simulink model "Simulation_DOA_rearanged_2020a"  (R2020a)
settings: Solver=ode4  StartTime=0.0  StopTime=0.03  RelTol=1e-3
values from neighbouring files (symbols this model uses):
  f_range = [20e3 45e3]    [Init.m]
  FFT_LENGTH = 256    [Init.m]
  noise_on_off = false    [Init.m]
  noise_type = 1    [Init.m]
  Sampling_rate = 256e3    (= 256000)    [Init.m]
undefined symbols (not defined in the file or in its folder): Coeff_han, runSim
libraries: dspsigops x29, dspsrcs4 x16, dsphdlmathfun x4, dsphdlxfrm x4, simulink x2, hdlsllib x1
(part 1 of 2)
settings Model: Creator=tigro  LastModifiedBy=franc
settings OptimizationCC: BlockReduction=off  ConditionallyExecuteInputs=off  DefaultParameterBehavior=Inlined
settings DebuggingCC: AlgebraicLoopMsg=error  ParameterOverflowMsg=none
settings HardwareCC: ProdBitPerPointer=32  ProdBitPerSizeT=32  ProdBitPerPtrDiffT=32  ProdLargestAtomicFloat=None  ProdIntDivRoundTo=Undefined  ProdEndianess=Unspecified  ProdWordSize=32  ProdHWDeviceType=ASIC/FPGA->ASIC/FPGA  TargetBitPerPointer=64  TargetBitPerSizeT=64  TargetBitPerPtrDiffT=64  TargetLongLongMode=on  TargetIntDivRoundTo=Zero  TargetEndianess=LittleEndian  TargetWordSize=64  TargetHWDeviceType=Custom Processor->MATLAB Host Computer  ProdEqTarget=off

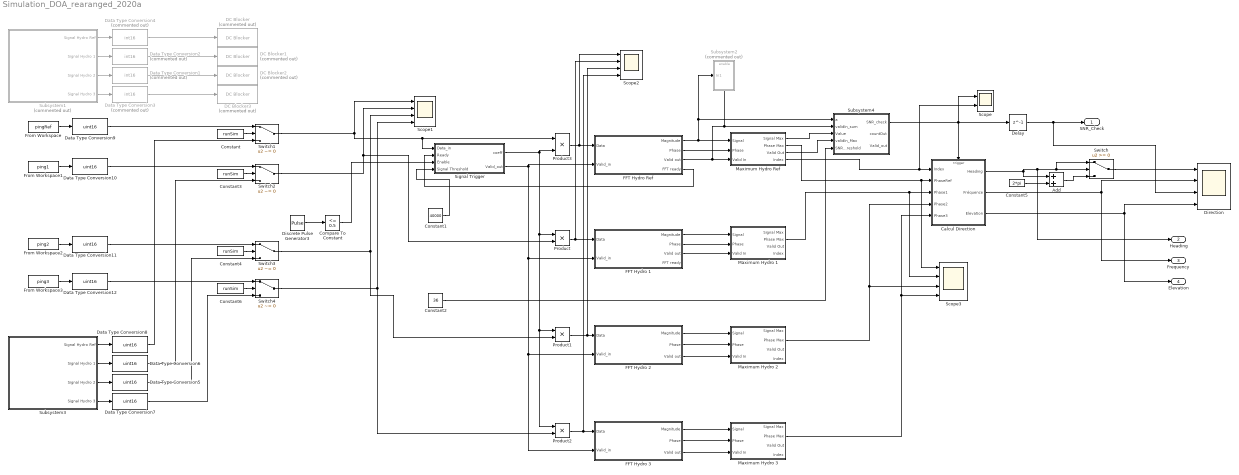
== system Simulation_DOA_rearanged_2020a ==
  Add : Sum
  Calcul Direction : Subsystem
  Compare To Constant : simulink/Logic and Bit Operations/Compare To Constant  relop=<=  const=0.5  OutDataTypeStr=boolean
  Constant{,3..4,6} (4 alike) : Constant  Value=runSim  SampleTime=-1
  Constant1 : Constant  Value=40000  OutDataTypeStr=uint16  SampleTime=-1
  Constant2 : Constant  Value=36  OutDataTypeStr=uint16  SampleTime=-1
  Constant5 : Constant  Value=2*pi
  DC Blocker{,1..3} (4 alike) : dspsigops/DC Blocker  Commented=on  Algorithm=FIR  NormalizedBandwidth=0.001  Length=50  Order=6  SimulateUsing=Code generation
      settings: SourceProductBaseCode=DS
  Data Type Conversion{1..4} (4 alike) : DataTypeConversion  Commented=on  OutMax=[4096]  OutDataTypeStr=int16
  Data Type Conversion{5..12} (8 alike) : DataTypeConversion  OutMax=[65535]  OutDataTypeStr=uint16
  Delay : Delay  DelayLength=1  InitialCondition=0
  Direction : Scope  NumInputPorts=4
  Discrete Pulse Generator3 : DiscretePulseGenerator  Period=512  PulseWidth=256  PhaseDelay=250  SampleTime=1/Sampling_rate
  FFT Hydro 1 : Subsystem
  FFT Hydro 2 : Subsystem
  FFT Hydro 3 : Subsystem
  FFT Hydro Ref : Subsystem
  From Workspace : FromWorkspace  VariableName=pingRef  SampleTime=1/Sampling_rate
  From Workspace1 : FromWorkspace  VariableName=ping1  SampleTime=1/Sampling_rate
  From Workspace2 : FromWorkspace  VariableName=ping2  SampleTime=1/Sampling_rate
  From Workspace3 : FromWorkspace  VariableName=ping3  SampleTime=1/Sampling_rate
  Maximum Hydro 1 : Subsystem
  Maximum Hydro 2 : Subsystem
  Maximum Hydro 3 : Subsystem
  Maximum Hydro Ref : Subsystem
  Product{,1..3} (4 alike) : Product
  Scope : Scope  NumInputPorts=2
  Scope1 : Scope  NumInputPorts=4
  Scope2 : Scope  NumInputPorts=4
  Scope3 : Scope  NumInputPorts=4
  Signal Trigger : Subsystem
  Subsystem1 : Subsystem  Commented=on
  Subsystem2 : Subsystem  Commented=on
  Subsystem3 : Subsystem
  Subsystem4 : Subsystem
  Switch : Switch
  Switch{1..4} (4 alike) : Switch  Criteria=u2 ~= 0
  SNR_Check : Outport
  Heading : Outport  Port=2
  Frequency : Outport  Port=3
  Elevation : Outport  Port=4
  wires:
  Maximum Hydro Ref/1(Signal Max) -> Subsystem4/3(" Value")
  Subsystem4/1(SNR_check) -> Delay/1, Scope/1, Calcul Direction/Trigger
  Maximum Hydro Ref/4(Index) -> Scope/2, Calcul Direction/1(Index)
  Calcul Direction/1(Heading) -> Heading/1, Switch/2, Switch/1, Add/1
  Add/1 -> Switch/3
  Constant5/1 -> Add/2
  Product3/1 -> Scope2/1, FFT Hydro Ref/1(Data)
  Product/1 -> Scope2/2, FFT Hydro 1/1(Data)
  Product1/1 -> Scope2/3, FFT Hydro 2/1(Data)
  Product2/1 -> Scope2/4, FFT Hydro 3/1(Data)
  FFT Hydro Ref/2(Phase) -> Maximum Hydro Ref/2(Phase)
  Maximum Hydro Ref/2(Phase Max) -> Scope3/1, Calcul Direction/2(PhaseRef)
  Maximum Hydro 1/2(Phase Max) -> Scope3/2, Calcul Direction/3(Phase1)
  Maximum Hydro 2/2(Phase Max) -> Calcul Direction/4(Phase2), Scope3/3
  Maximum Hydro 3/2(Phase Max) -> Calcul Direction/5(Phase3), Scope3/4
  Signal Trigger/2(Valid_out) -> FFT Hydro Ref/2(Valid_in), FFT Hydro 1/2(Valid_in), FFT Hydro 3/2(Valid_in), FFT Hydro 2/2(Valid_in)
  Signal Trigger/1(coeff) -> Product3/2, Product/1, Product1/1, Product2/1
  FFT Hydro 1/1(Magnitude) -> Maximum Hydro 1/1(Signal)
  FFT Hydro 1/2(Phase) -> Maximum Hydro 1/2(Phase)
  FFT Hydro 1/3(Valid out) -> Maximum Hydro 1/3(Valid In)
  FFT Hydro 2/1(Magnitude) -> Maximum Hydro 2/1(Signal)
  FFT Hydro 2/2(Phase) -> Maximum Hydro 2/2(Phase)
  FFT Hydro 2/3(Valid out) -> Maximum Hydro 2/3(Valid In)
  FFT Hydro 3/1(Magnitude) -> Maximum Hydro 3/1(Signal)
  FFT Hydro 3/2(Phase) -> Maximum Hydro 3/2(Phase)
  FFT Hydro 3/3(Valid out) -> Maximum Hydro 3/3(Valid In)
  Maximum Hydro Ref/3(Valid Out) -> Subsystem4/4(validIn_Max)
  FFT Hydro Ref/4(FFT ready) -> Signal Trigger/2(Ready)
  FFT Hydro Ref/3(Valid out) -> Maximum Hydro Ref/3(Valid In), Subsystem2/Enable, Subsystem4/2(validIn_sum)
  Calcul Direction/2(Fréquence) -> Frequency/1, Direction/2
  Switch/1 -> Direction/1
  FFT Hydro Ref/1(Magnitude) -> Maximum Hydro Ref/1(Signal), Subsystem2/1(In1), Subsystem4/1(a)
  Subsystem1/4(Signal Hydro 3) -> Data Type Conversion3/1
  Data Type Conversion3/1 -> DC Blocker3/1
  Data Type Conversion2/1 -> DC Blocker1/1
  Data Type Conversion4/1 -> DC Blocker/1
  Data Type Conversion1/1 -> DC Blocker2/1
  Subsystem1/2(Signal Hydro 1) -> Data Type Conversion2/1
  Subsystem1/3(Signal Hydro 2) -> Data Type Conversion1/1
  Subsystem1/1(Signal Hydro Ref) -> Data Type Conversion4/1
  Subsystem3/4(Signal Hydro 3) -> Data Type Conversion7/1
  Subsystem3/2(Signal Hydro 1) -> Data Type Conversion6/1
  Subsystem3/3(Signal Hydro 2) -> Data Type Conversion5/1
  Subsystem3/1(Signal Hydro Ref) -> Data Type Conversion8/1
  Switch2/1 -> Scope1/2, Product/2
  Switch3/1 -> Product1/2, Scope1/3
  Switch4/1 -> Product2/2, Scope1/4
  Discrete Pulse Generator3/1 -> Compare To Constant/1
  Switch1/1 -> Signal Trigger/1(Data_in), Product3/1, Scope1/1
  Delay/1 -> SNR_Check/1, Direction/3
  Compare To Constant/1 -> Signal Trigger/3(Enable)
  Constant1/1 -> Signal Trigger/4(Signal Threshold)
  Constant2/1 -> Subsystem4/5(SNR_Threshold)
  From Workspace/1 -> Data Type Conversion9/1
  From Workspace1/1 -> Data Type Conversion10/1
  From Workspace2/1 -> Data Type Conversion11/1
  From Workspace3/1 -> Data Type Conversion12/1
  Calcul Direction/3(Elevation) -> Elevation/1, Direction/4
  Data Type Conversion9/1 -> Switch1/1
  Data Type Conversion8/1 -> Switch1/3
  Data Type Conversion10/1 -> Switch2/1
  Data Type Conversion11/1 -> Switch3/1
  Data Type Conversion5/1 -> Switch3/3
  Data Type Conversion7/1 -> Switch4/3
  Data Type Conversion6/1 -> Switch2/3
  Data Type Conversion12/1 -> Switch4/1
  Constant/1 -> Switch1/2
  Constant3/1 -> Switch2/2
  Constant4/1 -> Switch3/2
  Constant6/1 -> Switch4/2

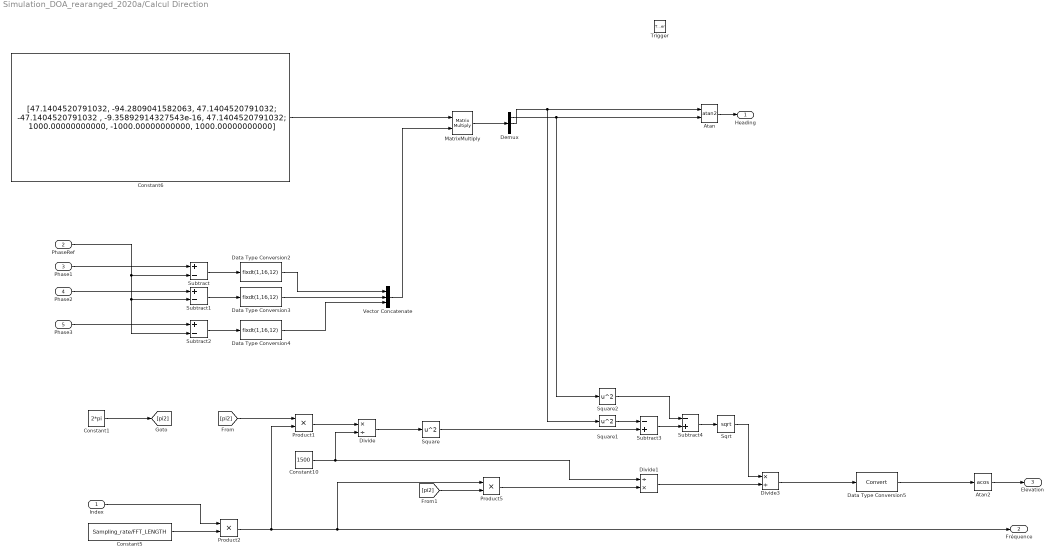
== system Simulation_DOA_rearanged_2020a/Calcul Direction ==
  Index : Inport
  PhaseRef : Inport  Port=2
  Phase1 : Inport  Port=3
  Phase2 : Inport  Port=4
  Phase3 : Inport  Port=5
  Trigger : TriggerPort  VariantControl=Variant  PortDimensions=1
  Atan : Trigonometry  Operator=atan2  ApproximationMethod=CORDIC  OutputSignalType=real
  Atan2 : Trigonometry  Operator=acos  ApproximationMethod=CORDIC  OutputSignalType=real
  Constant1 : Constant  Value=2*pi  OutDataTypeStr=fixdt(0,7,3)  SampleTime=-1
  Constant10 : Constant  Value=1500  OutDataTypeStr=fixdt(0,11)  SampleTime=-1
  Constant5 : Constant  Value=Sampling_rate/FFT_LENGTH  OutDataTypeStr=fixdt(0,10)  SampleTime=-1
  Constant6 : Constant  Value=|  VectorParams1D=off  OutDataTypeStr=fixdt(1,15,7)
      | [47.1404520791032,    -94.2809041582063,    47.1404520791032;
      | -47.1404520791032 ,   -9.35892914327543e-16,    47.1404520791032;
      | 1000.00000000000,   -1000.00000000000,    1000.00000000000]
  Data Type Conversion2 : DataTypeConversion  OutDataTypeStr=fixdt(1,16,12)
  Data Type Conversion3 : DataTypeConversion  OutDataTypeStr=fixdt(1,16,12)
  Data Type Conversion4 : DataTypeConversion  OutDataTypeStr=fixdt(1,16,12)
  Data Type Conversion5 : DataTypeConversion
  Demux : Demux  Outputs=3
  Divide : Product  Inputs=*/
  Divide1 : Product  Inputs=/*
  Divide3 : Product  Inputs=*/
  MatrixMultiply : Product  Multiplication=Matrix(*)
  Product1 : Product
  Product2 : Product
  Product5 : Product
  Sqrt : Sqrt  SaturateOnIntegerOverflow=on
  Square : Math  Operator=square  SignedPower=on  RndMeth=Zero  SaturateOnIntegerOverflow=on
  Square1 : Math  Operator=square  SignedPower=on  RndMeth=Zero  SaturateOnIntegerOverflow=on
  Square2 : Math  Operator=square  SignedPower=on  RndMeth=Zero  SaturateOnIntegerOverflow=on
  Subtract : Sum  Inputs=+-
  Subtract1 : Sum  Inputs=+-
  Subtract2 : Sum  Inputs=+-
  Subtract3 : Sum  Inputs=-+
  Subtract4 : Sum  Inputs=-+
  Vector Concatenate : Concatenate  NumInputs=3  Mode=Multidimensional array
  Heading : Outport  InitialOutput=0
  Fréquence : Outport  Port=2  InitialOutput=0
  Elevation : Outport  Port=3  InitialOutput=0
  wires:
  Vector Concatenate/1 -> MatrixMultiply/2
  Atan/1 -> Heading/1
  MatrixMultiply/1 -> Demux/1
  PhaseRef/1 -> Subtract/2, Subtract1/2, Subtract2/2
  Phase1/1 -> Subtract/1
  Phase2/1 -> Subtract1/1
  Phase3/1 -> Subtract2/1
  Subtract/1 -> Data Type Conversion2/1
  Subtract1/1 -> Data Type Conversion3/1
  Subtract2/1 -> Data Type Conversion4/1
  Constant6/1 -> MatrixMultiply/1
  Sqrt/1 -> Divide3/1
  Divide/1 -> Square/1
  [pi2] -> Product1/1
  Demux/2 -> Square1/1, Atan/1
  Constant1/1 -> [pi2]
  Divide1/1 -> Divide3/2
  Product5/1 -> Divide1/2
  [pi2] -> Product5/2
  Constant10/1 -> Divide/2, Divide1/1
  Subtract3/1 -> Subtract4/2
  Product1/1 -> Divide/1
  Square1/1 -> Subtract3/1
  Square/1 -> Subtract3/2
  Subtract4/1 -> Sqrt/1
  Constant5/1 -> Product2/2
  Index/1 -> Product2/1
  Square2/1 -> Subtract4/1
  Demux/1 -> Square2/1, Atan/2
  Divide3/1 -> Data Type Conversion5/1
  Product2/1 -> Fréquence/1, Product5/1, Product1/2
  Data Type Conversion2/1 -> Vector Concatenate/1
  Data Type Conversion3/1 -> Vector Concatenate/2
  Data Type Conversion4/1 -> Vector Concatenate/3
  Data Type Conversion5/1 -> Atan2/1
  Atan2/1 -> Elevation/1

== system Simulation_DOA_rearanged_2020a/FFT Hydro 1 ==
  Data : Inport
  Valid_in : Inport  Port=2
  Complex to Magnitude-Angle HDL Optimized : dsphdlmathfun/Complex to Magnitude-Angle HDL Optimized  NumIterationsSource=Property  NumIterations=CORDIC_Estimation  OutputFormat=Magnitude and angle  AngleFormat=Radians  ScaleOutput=on  SimulateUsing=Code generation
      settings: SourceProductBaseCode=DS
  FFT HDL Optimized : dsphdlxfrm/FFT HDL Optimized  FFTLength=FFT_LENGTH  Architecture=Burst Radix 2  ComplexMultiplication=Use 3 multipliers and 5 adders  BitReversedOutput=off  BitReversedInput=off  Normalize=on  SimulateUsing=Code generation  RoundingMethod=Floor  ResetInputPort=off  StartOutputPort=off  EndOutputPort=on
      settings: SourceProductBaseCode=DS
  Magnitude : Outport
  Phase : Outport  Port=2
  Valid out : Outport  Port=3
  FFT ready : Outport  Port=4
  wires:
  Valid_in/1 -> FFT HDL Optimized/2
  FFT HDL Optimized/1 -> Complex to Magnitude-Angle HDL Optimized/1
  Complex to Magnitude-Angle HDL Optimized/1 -> Magnitude/1
  Complex to Magnitude-Angle HDL Optimized/2 -> Phase/1
  Data/1 -> FFT HDL Optimized/1
  FFT HDL Optimized/3 -> Complex to Magnitude-Angle HDL Optimized/2
  Complex to Magnitude-Angle HDL Optimized/3 -> Valid out/1
  FFT HDL Optimized/4 -> FFT ready/1

== system Simulation_DOA_rearanged_2020a/FFT Hydro 2 ==
  Data : Inport
  Valid_in : Inport  Port=2
  Complex to Magnitude-Angle HDL Optimized : dsphdlmathfun/Complex to Magnitude-Angle HDL Optimized  NumIterationsSource=Property  NumIterations=CORDIC_Estimation  OutputFormat=Magnitude and angle  AngleFormat=Radians  ScaleOutput=on  SimulateUsing=Code generation
      settings: SourceProductBaseCode=DS
  FFT HDL Optimized : dsphdlxfrm/FFT HDL Optimized  FFTLength=FFT_LENGTH  Architecture=Burst Radix 2  ComplexMultiplication=Use 3 multipliers and 5 adders  BitReversedOutput=off  BitReversedInput=off  Normalize=on  SimulateUsing=Code generation  RoundingMethod=Floor  ResetInputPort=off  StartOutputPort=off  EndOutputPort=off
      settings: SourceProductBaseCode=DS
  Magnitude : Outport
  Phase : Outport  Port=2
  Valid out : Outport  Port=3
  wires:
  Valid_in/1 -> FFT HDL Optimized/2
  FFT HDL Optimized/1 -> Complex to Magnitude-Angle HDL Optimized/1
  FFT HDL Optimized/2 -> Complex to Magnitude-Angle HDL Optimized/2
  Complex to Magnitude-Angle HDL Optimized/1 -> Magnitude/1
  Complex to Magnitude-Angle HDL Optimized/3 -> Valid out/1
  Complex to Magnitude-Angle HDL Optimized/2 -> Phase/1
  Data/1 -> FFT HDL Optimized/1

== system Simulation_DOA_rearanged_2020a/FFT Hydro 3 ==
  Data : Inport
  Valid_in : Inport  Port=2
  Complex to Magnitude-Angle HDL Optimized : dsphdlmathfun/Complex to Magnitude-Angle HDL Optimized  NumIterationsSource=Property  NumIterations=CORDIC_Estimation  OutputFormat=Magnitude and angle  AngleFormat=Radians  ScaleOutput=on  SimulateUsing=Code generation
      settings: SourceProductBaseCode=DS
  FFT HDL Optimized : dsphdlxfrm/FFT HDL Optimized  FFTLength=FFT_LENGTH  Architecture=Burst Radix 2  ComplexMultiplication=Use 3 multipliers and 5 adders  BitReversedOutput=off  BitReversedInput=off  Normalize=on  SimulateUsing=Code generation  RoundingMethod=Floor  ResetInputPort=off  StartOutputPort=off  EndOutputPort=off
      settings: SourceProductBaseCode=DS
  Magnitude : Outport
  Phase : Outport  Port=2
  Valid out : Outport  Port=3
  wires:
  Valid_in/1 -> FFT HDL Optimized/2
  FFT HDL Optimized/1 -> Complex to Magnitude-Angle HDL Optimized/1
  FFT HDL Optimized/2 -> Complex to Magnitude-Angle HDL Optimized/2
  Complex to Magnitude-Angle HDL Optimized/1 -> Magnitude/1
  Complex to Magnitude-Angle HDL Optimized/3 -> Valid out/1
  Complex to Magnitude-Angle HDL Optimized/2 -> Phase/1
  Data/1 -> FFT HDL Optimized/1

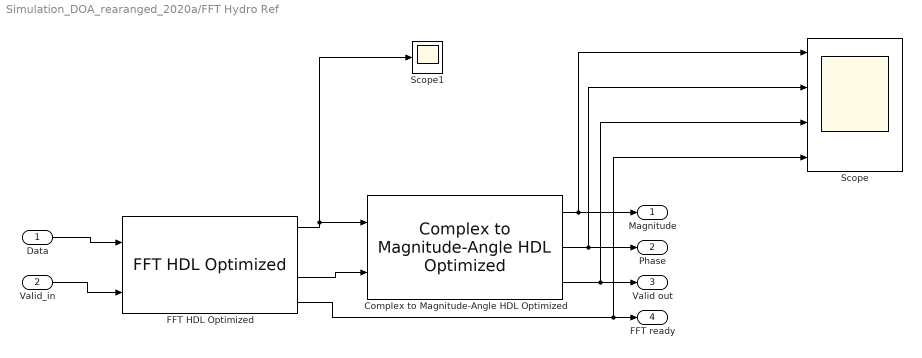
== system Simulation_DOA_rearanged_2020a/FFT Hydro Ref ==
  Data : Inport
  Valid_in : Inport  Port=2
  Complex to Magnitude-Angle HDL Optimized : dsphdlmathfun/Complex to Magnitude-Angle HDL Optimized  NumIterationsSource=Property  NumIterations=CORDIC_Estimation  OutputFormat=Magnitude and angle  AngleFormat=Radians  ScaleOutput=on  SimulateUsing=Code generation
      settings: SourceProductBaseCode=DS
  FFT HDL Optimized : dsphdlxfrm/FFT HDL Optimized  FFTLength=FFT_LENGTH  Architecture=Burst Radix 2  ComplexMultiplication=Use 3 multipliers and 5 adders  BitReversedOutput=off  BitReversedInput=off  Normalize=on  SimulateUsing=Code generation  RoundingMethod=Floor  ResetInputPort=off  StartOutputPort=off  EndOutputPort=on
      settings: SourceProductBaseCode=DS
  Scope : Scope  NumInputPorts=4
  Scope1 : Scope
  Magnitude : Outport
  Phase : Outport  Port=2
  Valid out : Outport  Port=3
  FFT ready : Outport  Port=4
  wires:
  Valid_in/1 -> FFT HDL Optimized/2
  FFT HDL Optimized/1 -> Complex to Magnitude-Angle HDL Optimized/1, Scope1/1
  Complex to Magnitude-Angle HDL Optimized/1 -> Scope/1, Magnitude/1
  Complex to Magnitude-Angle HDL Optimized/2 -> Scope/2, Phase/1
  Data/1 -> FFT HDL Optimized/1
  FFT HDL Optimized/3 -> Complex to Magnitude-Angle HDL Optimized/2
  Complex to Magnitude-Angle HDL Optimized/3 -> Scope/3, Valid out/1
  FFT HDL Optimized/4 -> Scope/4, FFT ready/1

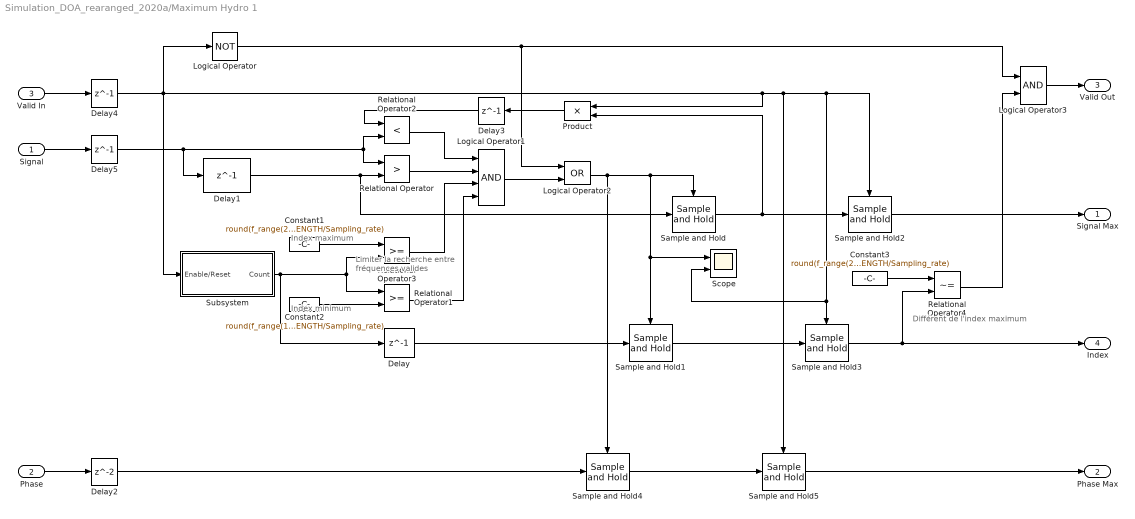
== system Simulation_DOA_rearanged_2020a/Maximum Hydro 1 ==
  note: Index minimum
  note: Index maximum
  note: Limiter la recherche
      | entre fréquences valides
  note: Différent de l'index
      | maximum
  Signal : Inport
  Phase : Inport  Port=2
  Valid In : Inport  Port=3
  Constant1 : Constant  Value=round(f_range(2)*FFT_LENGTH/Sampling_rate)  OutDataTypeStr=fixdt(0,6)  SampleTime=1/Sampling_rate
  Constant2 : Constant  Value=round(f_range(1)*FFT_LENGTH/Sampling_rate)  OutDataTypeStr=fixdt(0,6)  SampleTime=1/Sampling_rate
  Constant3 : Constant  Value=round(f_range(2)*FFT_LENGTH/Sampling_rate)  OutDataTypeStr=fixdt(0,6)  SampleTime=1/Sampling_rate
  Delay : Delay  DelayLength=1  InitialCondition=0
  Delay{1,3..5} (4 alike) : Delay  DelayLength=1  InitialCondition=0  UseCircularBuffer=on
  Delay2 : Delay  InitialCondition=0  UseCircularBuffer=on
  Logical Operator : Logic  Operator=NOT  IconShape=distinctive  AllPortsSameDT=off  OutDataTypeStr=boolean
  Logical Operator1 : Logic  Inputs=4  AllPortsSameDT=off  OutDataTypeStr=boolean
  Logical Operator2 : Logic  Operator=OR  AllPortsSameDT=off  OutDataTypeStr=boolean
  Logical Operator3 : Logic  AllPortsSameDT=off  OutDataTypeStr=boolean
  Product : Product
  Relational Operator : RelationalOperator  Operator=>  OutDataTypeStr=boolean  RndMeth=Nearest
  Relational Operator1 : RelationalOperator  OutDataTypeStr=boolean  RndMeth=Nearest
  Relational Operator2 : RelationalOperator  Operator=<  OutDataTypeStr=boolean  RndMeth=Nearest
  Relational Operator3 : RelationalOperator  OutDataTypeStr=boolean  RndMeth=Nearest
  Relational Operator4 : RelationalOperator  Operator=~=  OutDataTypeStr=boolean  RndMeth=Nearest
  Sample and Hold{,1..5} (6 alike) : dspsigops/Sample and Hold  trig=Falling edge  initCond=0  latchinput=off
  Scope : Scope  NumInputPorts=2
  Subsystem : Subsystem
  Signal Max : Outport  VectorParamsAs1DForOutWhenUnconnected=off
  Phase Max : Outport  Port=2  VectorParamsAs1DForOutWhenUnconnected=off
  Valid Out : Outport  Port=3  VectorParamsAs1DForOutWhenUnconnected=off
  Index : Outport  Port=4  VectorParamsAs1DForOutWhenUnconnected=off
  wires:
  Sample and Hold/1 -> Sample and Hold2/1, Product/2
  Signal/1 -> Delay5/1
  Sample and Hold1/1 -> Sample and Hold3/1
  Valid In/1 -> Delay4/1
  Delay1/1 -> Sample and Hold/1, Relational Operator/2
  Sample and Hold2/1 -> Signal Max/1
  Constant2/1 -> Relational Operator1/2
  Sample and Hold4/1 -> Sample and Hold5/1
  Phase/1 -> Delay2/1
  Sample and Hold5/1 -> Phase Max/1
  Subsystem/1(Count) -> Delay/1, Relational Operator1/1, Relational Operator3/2
  Relational Operator2/1 -> Logical Operator1/1
  Relational Operator/1 -> Logical Operator1/2
  Delay3/1 -> Relational Operator2/1
  Product/1 -> Delay3/1
  Delay4/1 -> Logical Operator/1, Sample and Hold2/Trigger, Sample and Hold3/Trigger, Scope/2, Sample and Hold5/Trigger, Product/1, Subsystem/1(Enable/Reset)
  Delay5/1 -> Relational Operator2/2, Relational Operator/1, Delay1/1
  Delay2/1 -> Sample and Hold4/1
  Constant1/1 -> Relational Operator3/1
  Relational Operator1/1 -> Logical Operator1/4
  Logical Operator/1 -> Logical Operator2/1, Logical Operator3/1
  Logical Operator3/1 -> Valid Out/1
  Relational Operator3/1 -> Logical Operator1/3
  Relational Operator4/1 -> Logical Operator3/2
  Sample and Hold3/1 -> Index/1, Relational Operator4/2
  Constant3/1 -> Relational Operator4/1
  Logical Operator1/1 -> Logical Operator2/2
  Logical Operator2/1 -> Sample and Hold4/Trigger, Sample and Hold/Trigger, Scope/1, Sample and Hold1/Trigger
  Delay/1 -> Sample and Hold1/1

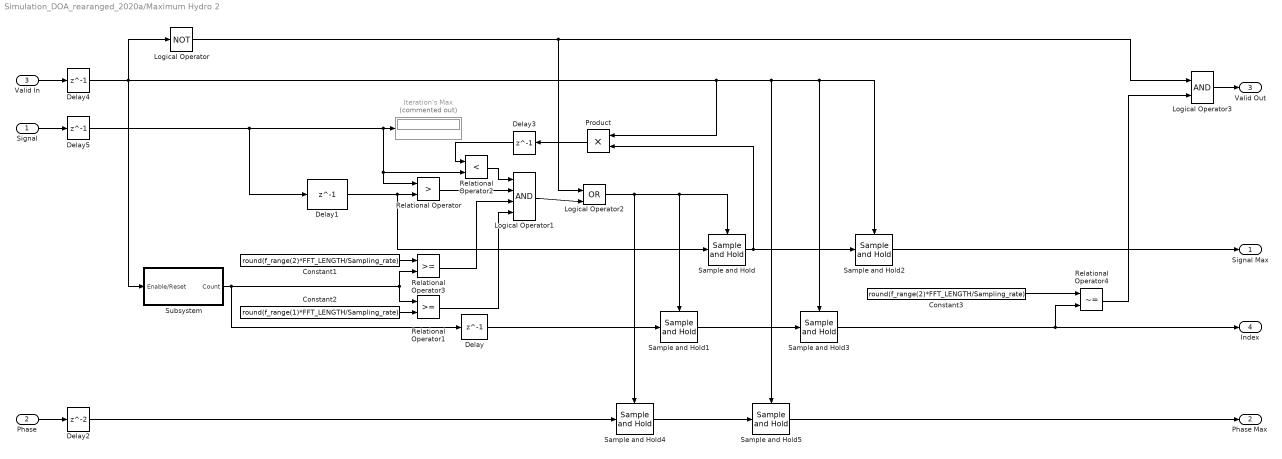
== system Simulation_DOA_rearanged_2020a/Maximum Hydro 2 ==
  Signal : Inport
  Phase : Inport  Port=2
  Valid In : Inport  Port=3
  Constant1 : Constant  Value=round(f_range(2)*FFT_LENGTH/Sampling_rate)  OutDataTypeStr=fixdt(0,6)  SampleTime=1/Sampling_rate
  Constant2 : Constant  Value=round(f_range(1)*FFT_LENGTH/Sampling_rate)  OutDataTypeStr=fixdt(0,6)  SampleTime=1/Sampling_rate
  Constant3 : Constant  Value=round(f_range(2)*FFT_LENGTH/Sampling_rate)  OutDataTypeStr=fixdt(0,6)  SampleTime=1/Sampling_rate
  Delay : Delay  DelayLength=1  InitialCondition=0
  Delay{1,3..5} (4 alike) : Delay  DelayLength=1  InitialCondition=0  UseCircularBuffer=on
  Delay2 : Delay  InitialCondition=0  UseCircularBuffer=on
  Iteration's Max : Display  Commented=on
  Logical Operator : Logic  Operator=NOT  IconShape=distinctive  AllPortsSameDT=off  OutDataTypeStr=boolean
  Logical Operator1 : Logic  Inputs=4  AllPortsSameDT=off  OutDataTypeStr=boolean
  Logical Operator2 : Logic  Operator=OR  IconShape=distinctive  AllPortsSameDT=off  OutDataTypeStr=boolean
  Logical Operator3 : Logic  AllPortsSameDT=off  OutDataTypeStr=boolean
  Product : Product
  Relational Operator : RelationalOperator  Operator=>  OutDataTypeStr=boolean  RndMeth=Nearest
  Relational Operator1 : RelationalOperator  OutDataTypeStr=boolean  RndMeth=Nearest
  Relational Operator2 : RelationalOperator  Operator=<  OutDataTypeStr=boolean  RndMeth=Nearest
  Relational Operator3 : RelationalOperator  OutDataTypeStr=boolean  RndMeth=Nearest
  Relational Operator4 : RelationalOperator  Operator=~=  OutDataTypeStr=boolean  RndMeth=Nearest
  Sample and Hold{,1..5} (6 alike) : dspsigops/Sample and Hold  trig=Falling edge  initCond=0  latchinput=off
  Subsystem : Subsystem
  Signal Max : Outport  VectorParamsAs1DForOutWhenUnconnected=off
  Phase Max : Outport  Port=2  VectorParamsAs1DForOutWhenUnconnected=off
  Valid Out : Outport  Port=3  VectorParamsAs1DForOutWhenUnconnected=off
  Index : Outport  Port=4  VectorParamsAs1DForOutWhenUnconnected=off
  wires:
  Sample and Hold/1 -> Sample and Hold2/1, Product/2
  Signal/1 -> Delay5/1
  Sample and Hold1/1 -> Sample and Hold3/1
  Valid In/1 -> Delay4/1
  Delay1/1 -> Sample and Hold/1, Relational Operator/2
  Sample and Hold2/1 -> Signal Max/1
  Constant2/1 -> Relational Operator1/2
  Sample and Hold4/1 -> Sample and Hold5/1
  Phase/1 -> Delay2/1
  Sample and Hold5/1 -> Phase Max/1
  Subsystem/1(Count) -> Relational Operator1/1, Relational Operator3/2, Delay/1
  Relational Operator2/1 -> Logical Operator1/1
  Relational Operator/1 -> Logical Operator1/2
  Delay3/1 -> Relational Operator2/1
  Product/1 -> Delay3/1
  Delay4/1 -> Logical Operator/1, Product/1, Sample and Hold2/Trigger, Sample and Hold3/Trigger, Sample and Hold5/Trigger, Subsystem/1(Enable/Reset)
  Delay5/1 -> Relational Operator/1, Relational Operator2/2, Iteration's Max/1, Delay1/1
  Delay2/1 -> Sample and Hold4/1
  Constant1/1 -> Relational Operator3/1
  Relational Operator1/1 -> Logical Operator1/4
  Logical Operator/1 -> Logical Operator3/1, Logical Operator2/1
  Logical Operator3/1 -> Valid Out/1
  Relational Operator3/1 -> Logical Operator1/3
  Relational Operator4/1 -> Logical Operator3/2
  Sample and Hold3/1 -> Index/1, Relational Operator4/2
  Constant3/1 -> Relational Operator4/1
  Logical Operator1/1 -> Logical Operator2/2
  Logical Operator2/1 -> Sample and Hold/Trigger, Sample and Hold1/Trigger, Sample and Hold4/Trigger
  Delay/1 -> Sample and Hold1/1

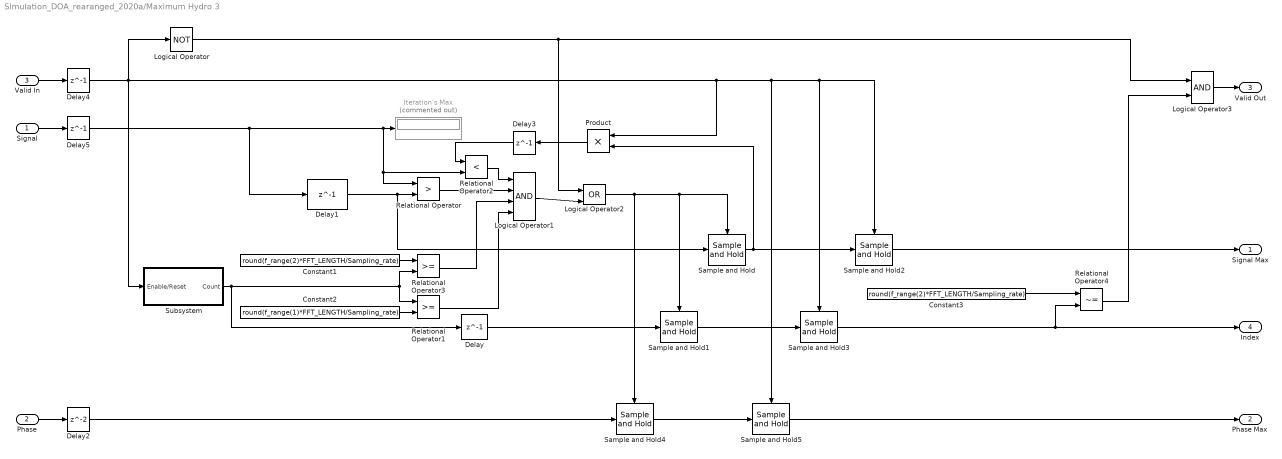
== system Simulation_DOA_rearanged_2020a/Maximum Hydro 3 ==
  Signal : Inport
  Phase : Inport  Port=2
  Valid In : Inport  Port=3
  Constant1 : Constant  Value=round(f_range(2)*FFT_LENGTH/Sampling_rate)  OutDataTypeStr=fixdt(0,6)  SampleTime=1/Sampling_rate
  Constant2 : Constant  Value=round(f_range(1)*FFT_LENGTH/Sampling_rate)  OutDataTypeStr=fixdt(0,6)  SampleTime=1/Sampling_rate
  Constant3 : Constant  Value=round(f_range(2)*FFT_LENGTH/Sampling_rate)  OutDataTypeStr=fixdt(0,6)  SampleTime=1/Sampling_rate
  Delay : Delay  DelayLength=1  InitialCondition=0
  Delay{1,3..5} (4 alike) : Delay  DelayLength=1  InitialCondition=0  UseCircularBuffer=on
  Delay2 : Delay  InitialCondition=0  UseCircularBuffer=on
  Iteration's Max : Display  Commented=on
  Logical Operator : Logic  Operator=NOT  IconShape=distinctive  AllPortsSameDT=off  OutDataTypeStr=boolean
  Logical Operator1 : Logic  Inputs=4  AllPortsSameDT=off  OutDataTypeStr=boolean
  Logical Operator2 : Logic  Operator=OR  IconShape=distinctive  AllPortsSameDT=off  OutDataTypeStr=boolean
  Logical Operator3 : Logic  AllPortsSameDT=off  OutDataTypeStr=boolean
  Product : Product
  Relational Operator : RelationalOperator  Operator=>  OutDataTypeStr=boolean  RndMeth=Nearest
  Relational Operator1 : RelationalOperator  OutDataTypeStr=boolean  RndMeth=Nearest
  Relational Operator2 : RelationalOperator  Operator=<  OutDataTypeStr=boolean  RndMeth=Nearest
  Relational Operator3 : RelationalOperator  OutDataTypeStr=boolean  RndMeth=Nearest
  Relational Operator4 : RelationalOperator  Operator=~=  OutDataTypeStr=boolean  RndMeth=Nearest
  Sample and Hold{,1..5} (6 alike) : dspsigops/Sample and Hold  trig=Falling edge  initCond=0  latchinput=off
  Subsystem : Subsystem
  Signal Max : Outport  VectorParamsAs1DForOutWhenUnconnected=off
  Phase Max : Outport  Port=2  VectorParamsAs1DForOutWhenUnconnected=off
  Valid Out : Outport  Port=3  VectorParamsAs1DForOutWhenUnconnected=off
  Index : Outport  Port=4  VectorParamsAs1DForOutWhenUnconnected=off
  wires:
  Sample and Hold/1 -> Sample and Hold2/1, Product/2
  Signal/1 -> Delay5/1
  Sample and Hold1/1 -> Sample and Hold3/1
  Valid In/1 -> Delay4/1
  Delay1/1 -> Sample and Hold/1, Relational Operator/2
  Sample and Hold2/1 -> Signal Max/1
  Constant2/1 -> Relational Operator1/2
  Sample and Hold4/1 -> Sample and Hold5/1
  Phase/1 -> Delay2/1
  Sample and Hold5/1 -> Phase Max/1
  Subsystem/1(Count) -> Relational Operator1/1, Relational Operator3/2, Delay/1
  Relational Operator2/1 -> Logical Operator1/1
  Relational Operator/1 -> Logical Operator1/2
  Delay3/1 -> Relational Operator2/1
  Product/1 -> Delay3/1
  Delay4/1 -> Logical Operator/1, Product/1, Sample and Hold2/Trigger, Sample and Hold3/Trigger, Sample and Hold5/Trigger, Subsystem/1(Enable/Reset)
  Delay5/1 -> Relational Operator/1, Relational Operator2/2, Iteration's Max/1, Delay1/1
  Delay2/1 -> Sample and Hold4/1
  Constant1/1 -> Relational Operator3/1
  Relational Operator1/1 -> Logical Operator1/4
  Logical Operator/1 -> Logical Operator3/1, Logical Operator2/1
  Logical Operator3/1 -> Valid Out/1
  Relational Operator3/1 -> Logical Operator1/3
  Relational Operator4/1 -> Logical Operator3/2
  Sample and Hold3/1 -> Index/1, Relational Operator4/2
  Constant3/1 -> Relational Operator4/1
  Logical Operator1/1 -> Logical Operator2/2
  Logical Operator2/1 -> Sample and Hold/Trigger, Sample and Hold1/Trigger, Sample and Hold4/Trigger
  Delay/1 -> Sample and Hold1/1

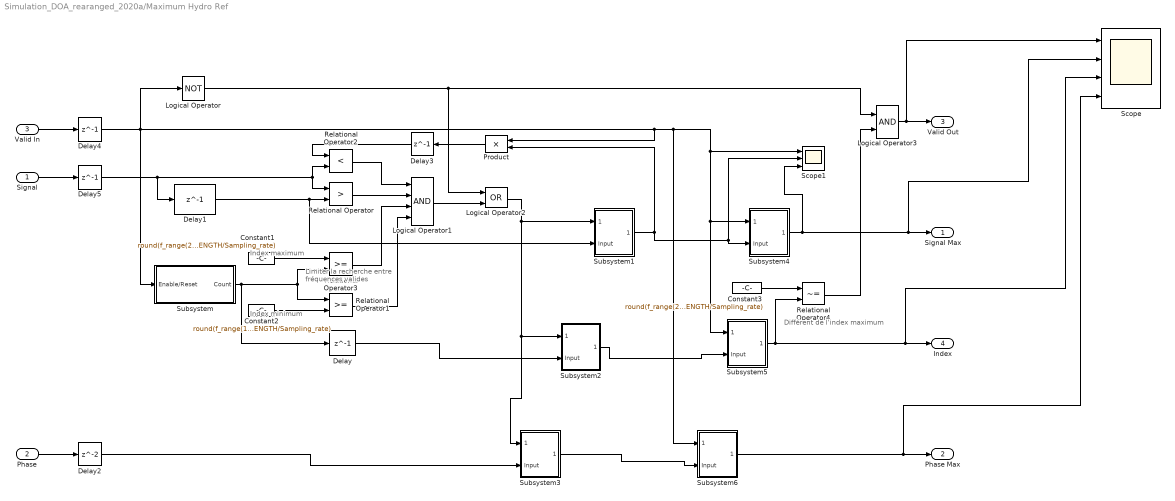
== system Simulation_DOA_rearanged_2020a/Maximum Hydro Ref ==
  note: Index minimum
  note: Index maximum
  note: Limiter la recherche
      | entre fréquences valides
  note: Différent de l'index
      | maximum
  Signal : Inport
  Phase : Inport  Port=2
  Valid In : Inport  Port=3
  Constant1 : Constant  Value=round(f_range(2)*FFT_LENGTH/Sampling_rate)  OutDataTypeStr=fixdt(0,6)  SampleTime=1/Sampling_rate
  Constant2 : Constant  Value=round(f_range(1)*FFT_LENGTH/Sampling_rate)  OutDataTypeStr=fixdt(0,6)  SampleTime=1/Sampling_rate
  Constant3 : Constant  Value=round(f_range(2)*FFT_LENGTH/Sampling_rate)  OutDataTypeStr=fixdt(0,6)  SampleTime=1/Sampling_rate
  Delay : Delay  DelayLength=1  InitialCondition=0
  Delay{1,3..5} (4 alike) : Delay  DelayLength=1  InitialCondition=0  UseCircularBuffer=on
  Delay2 : Delay  InitialCondition=0  UseCircularBuffer=on
  Logical Operator : Logic  Operator=NOT  IconShape=distinctive  AllPortsSameDT=off  OutDataTypeStr=boolean
  Logical Operator1 : Logic  Inputs=4  AllPortsSameDT=off  OutDataTypeStr=boolean
  Logical Operator2 : Logic  Operator=OR  AllPortsSameDT=off  OutDataTypeStr=boolean
  Logical Operator3 : Logic  AllPortsSameDT=off  OutDataTypeStr=boolean
  Product : Product
  Relational Operator : RelationalOperator  Operator=>  OutDataTypeStr=boolean  RndMeth=Nearest
  Relational Operator1 : RelationalOperator  OutDataTypeStr=boolean  RndMeth=Nearest
  Relational Operator2 : RelationalOperator  Operator=<  OutDataTypeStr=boolean  RndMeth=Nearest
  Relational Operator3 : RelationalOperator  OutDataTypeStr=boolean  RndMeth=Nearest
  Relational Operator4 : RelationalOperator  Operator=~=  OutDataTypeStr=boolean  RndMeth=Nearest
  Scope : Scope  NumInputPorts=4
  Scope1 : Scope  NumInputPorts=3
  Subsystem : Subsystem
  Subsystem1 : Subsystem  TreatAsAtomicUnit=on
  Subsystem2 : Subsystem  TreatAsAtomicUnit=on
  Subsystem3 : Subsystem  TreatAsAtomicUnit=on
  Subsystem4 : Subsystem  TreatAsAtomicUnit=on
  Subsystem5 : Subsystem  TreatAsAtomicUnit=on
  Subsystem6 : Subsystem  TreatAsAtomicUnit=on
  Signal Max : Outport  VectorParamsAs1DForOutWhenUnconnected=off
  Phase Max : Outport  Port=2  VectorParamsAs1DForOutWhenUnconnected=off
  Valid Out : Outport  Port=3  VectorParamsAs1DForOutWhenUnconnected=off
  Index : Outport  Port=4  VectorParamsAs1DForOutWhenUnconnected=off
  wires:
  Subsystem1/1(" ") -> Product/2, Subsystem4/2(Input), Scope1/2
  Signal/1 -> Delay5/1
  Subsystem2/1(" ") -> Subsystem5/2(Input)
  Valid In/1 -> Delay4/1
  Delay1/1 -> Subsystem1/2(Input), Relational Operator/2
  Subsystem4/1(" ") -> Scope1/3, Scope/2, Signal Max/1
  Constant2/1 -> Relational Operator1/2
  Subsystem3/1(" ") -> Subsystem6/2(Input)
  Phase/1 -> Delay2/1
  Subsystem6/1(" ") -> Phase Max/1, Scope/4
  Subsystem/1(Count) -> Delay/1, Relational Operator1/1, Relational Operator3/2
  Relational Operator2/1 -> Logical Operator1/1
  Relational Operator/1 -> Logical Operator1/2
  Delay3/1 -> Relational Operator2/1
  Product/1 -> Delay3/1
  Delay4/1 -> Logical Operator/1, Subsystem6/1(Trigger), Subsystem5/1(Trigger), Subsystem4/1(Trigger), Scope1/1, Product/1, Subsystem/1(Enable/Reset)
  Delay5/1 -> Relational Operator2/2, Relational Operator/1, Delay1/1
  Delay2/1 -> Subsystem3/2(Input)
  Constant1/1 -> Relational Operator3/1
  Relational Operator1/1 -> Logical Operator1/4
  Logical Operator/1 -> Logical Operator2/1, Logical Operator3/1
  Logical Operator3/1 -> Scope/1, Valid Out/1
  Relational Operator3/1 -> Logical Operator1/3
  Relational Operator4/1 -> Logical Operator3/2
  Constant3/1 -> Relational Operator4/1
  Logical Operator1/1 -> Logical Operator2/2
  Logical Operator2/1 -> Subsystem1/1(Trigger), Subsystem3/1(Trigger), Subsystem2/1(Trigger)
  Delay/1 -> Subsystem2/2(Input)
  Subsystem5/1(" ") -> Index/1, Scope/3, Relational Operator4/2

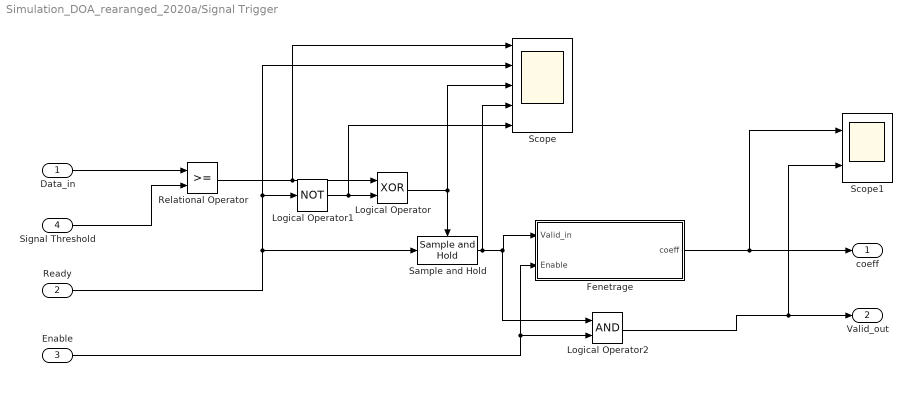
== system Simulation_DOA_rearanged_2020a/Signal Trigger ==
  Data_in : Inport
  Ready : Inport  Port=2  OutDataTypeStr=boolean
  Enable : Inport  Port=3  OutDataTypeStr=boolean
  Signal Threshold : Inport  Port=4
  Fenetrage : Subsystem
  Logical Operator : Logic  Operator=XOR  AllPortsSameDT=off  OutDataTypeStr=boolean
  Logical Operator1 : Logic  Operator=NOT  IconShape=distinctive  AllPortsSameDT=off  OutDataTypeStr=boolean
  Logical Operator2 : Logic  AllPortsSameDT=off  OutDataTypeStr=boolean
  Relational Operator : RelationalOperator  OutDataTypeStr=boolean  RndMeth=Nearest
  Sample and Hold : dspsigops/Sample and Hold  trig=Rising edge  initCond=0  latchinput=off
  Scope : Scope  NumInputPorts=5
  Scope1 : Scope  NumInputPorts=2
  coeff : Outport
  Valid_out : Outport  Port=2
  wires:
  Data_in/1 -> Relational Operator/1
  Fenetrage/1(coeff) -> Scope1/1, coeff/1
  Relational Operator/1 -> Logical Operator/1, Scope/1
  Ready/1 -> Scope/2, Logical Operator1/1, Sample and Hold/1
  Logical Operator/1 -> Scope/3, Sample and Hold/Trigger
  Sample and Hold/1 -> Logical Operator2/1, Fenetrage/1(Valid_in), Scope/4
  Logical Operator1/1 -> Scope/5, Logical Operator/2
  Enable/1 -> Logical Operator2/2, Fenetrage/2(Enable)
  Logical Operator2/1 -> Scope1/2, Valid_out/1
  Signal Threshold/1 -> Relational Operator/2

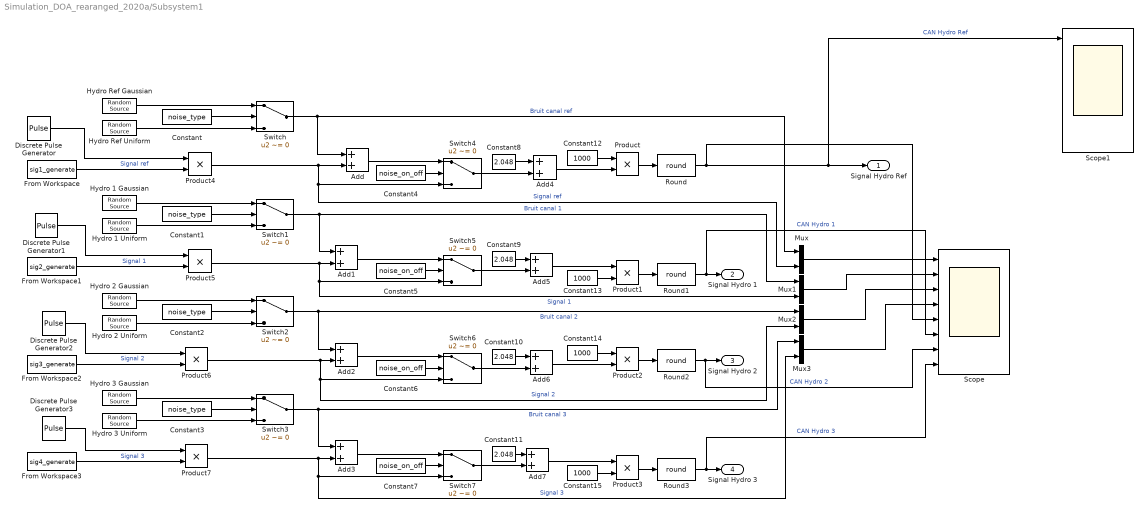
== system Simulation_DOA_rearanged_2020a/Subsystem1 ==
  Add{,1..7} (8 alike) : Sum
  Constant{,1..3} (4 alike) : Constant  Value=noise_type  VectorParams1D=off  SampleTime=-1
  Constant{8..11} (4 alike) : Constant  Value=2.048  VectorParams1D=off  SampleTime=-1
  Constant{12..15} (4 alike) : Constant  Value=1000  VectorParams1D=off  SampleTime=-1
  Constant{4..7} (4 alike) : Constant  Value=noise_on_off  VectorParams1D=off  SampleTime=-1
  Discrete Pulse Generator{,1..3} (4 alike) : DiscretePulseGenerator  Period=128  PulseWidth=50  SampleTime=1/Sampling_rate
  From Workspace : FromWorkspace  VariableName=sig1_generate  SampleTime=1/Sampling_rate
  From Workspace1 : FromWorkspace  VariableName=sig2_generate  SampleTime=1/Sampling_rate
  From Workspace2 : FromWorkspace  VariableName=sig3_generate  SampleTime=1/Sampling_rate
  From Workspace3 : FromWorkspace  VariableName=sig4_generate  SampleTime=1/Sampling_rate
  Hydro 1 Gaussian : dspsrcs4/Random Source  SrcType=Gaussian  NormMethod=Ziggurat  CltLength=12  MinVal=0  MaxVal=1  MeanVal=0  VarVal=variance  RepMode=Specify seed  rawSeed=randSeed2  IsInherit=off  SampMode=Discrete  SampTime=1/Sampling_rate  SampFrame=1  DataType=Double  OutComplex=Real  OutputFrames=off
  Hydro 1 Uniform : dspsrcs4/Random Source  SrcType=Uniform  NormMethod=Ziggurat  CltLength=12  MinVal=-0.9  MaxVal=0.9  MeanVal=0  VarVal=1  RepMode=Specify seed  rawSeed=4948745  IsInherit=off  SampMode=Discrete  SampTime=1/Sampling_rate  SampFrame=1  DataType=Double  OutComplex=Real  OutputFrames=off
  Hydro 2 Gaussian : dspsrcs4/Random Source  SrcType=Gaussian  NormMethod=Ziggurat  CltLength=12  MinVal=0  MaxVal=1  MeanVal=0  VarVal=variance  RepMode=Specify seed  rawSeed=randSeed3  IsInherit=off  SampMode=Discrete  SampTime=1/Sampling_rate  SampFrame=1  DataType=Double  OutComplex=Real  OutputFrames=off
  Hydro 2 Uniform : dspsrcs4/Random Source  SrcType=Uniform  NormMethod=Ziggurat  CltLength=12  MinVal=-0.9  MaxVal=0.9  MeanVal=0  VarVal=1  RepMode=Specify seed  rawSeed=2398385  IsInherit=off  SampMode=Discrete  SampTime=1/Sampling_rate  SampFrame=1  DataType=Double  OutComplex=Real  OutputFrames=off
  Hydro 3 Gaussian : dspsrcs4/Random Source  SrcType=Gaussian  NormMethod=Ziggurat  CltLength=12  MinVal=0  MaxVal=1  MeanVal=0  VarVal=variance  RepMode=Specify seed  rawSeed=randSeed4  IsInherit=off  SampMode=Discrete  SampTime=1/Sampling_rate  SampFrame=1  DataType=Double  OutComplex=Real  OutputFrames=off
  Hydro 3 Uniform : dspsrcs4/Random Source  SrcType=Uniform  NormMethod=Ziggurat  CltLength=12  MinVal=-0.9  MaxVal=0.9  MeanVal=0  VarVal=1  RepMode=Specify seed  rawSeed=9274563  IsInherit=off  SampMode=Discrete  SampTime=1/Sampling_rate  SampFrame=1  DataType=Double  OutComplex=Real  OutputFrames=off
  Hydro Ref Gaussian : dspsrcs4/Random Source  SrcType=Gaussian  NormMethod=Ziggurat  CltLength=12  MinVal=0  MaxVal=1  MeanVal=0  VarVal=variance  RepMode=Specify seed  rawSeed=randSeed1  IsInherit=off  SampMode=Discrete  SampTime=1/Sampling_rate  SampFrame=1  DataType=Double  OutComplex=Real  OutputFrames=off
  Hydro Ref Uniform : dspsrcs4/Random Source  SrcType=Uniform  NormMethod=Ziggurat  CltLength=12  MinVal=-0.9  MaxVal=0.9  MeanVal=0  VarVal=1  RepMode=Specify seed  rawSeed=3409859  IsInherit=off  SampMode=Discrete  SampTime=1/Sampling_rate  SampFrame=1  DataType=Double  OutComplex=Real  OutputFrames=off
  Mux{,1..3} (4 alike) : Mux  Inputs=2
  Product{,1..7} (8 alike) : Product
  Round{,1..3} (4 alike) : Rounding  Operator=round
  Scope : Scope  NumInputPorts=8
  Scope1 : Scope  NumInputPorts=8
  Switch{,1..7} (8 alike) : Switch  Criteria=u2 ~= 0
  Signal Hydro Ref : Outport
  Signal Hydro 1 : Outport  Port=2
  Signal Hydro 2 : Outport  Port=3
  Signal Hydro 3 : Outport  Port=4
  wires:
  Hydro Ref Uniform/1 -> Switch/3
  Hydro Ref Gaussian/1 -> Switch/1
  Product4/1 -> Switch4/3, Mux/2, Add/2  "Signal ref"
  Switch/1 -> Add/1, Mux/1  "Bruit canal ref"
  Constant/1 -> Switch/2
  Hydro 1 Uniform/1 -> Switch1/3
  Hydro 1 Gaussian/1 -> Switch1/1
  Constant1/1 -> Switch1/2
  Product5/1 -> Switch5/3, Mux1/2, Add1/2  "Signal 1"
  Switch2/1 -> Add2/1, Mux2/1  "Bruit canal 2"
  Hydro 2 Uniform/1 -> Switch2/3
  Hydro 2 Gaussian/1 -> Switch2/1
  Constant2/1 -> Switch2/2
  Product6/1 -> Switch6/3, Mux2/2, Add2/2  "Signal 2"
  Switch3/1 -> Mux3/1, Add3/1  "Bruit canal 3"
  Hydro 3 Uniform/1 -> Switch3/3
  Hydro 3 Gaussian/1 -> Switch3/1
  Constant3/1 -> Switch3/2
  Product7/1 -> Mux3/2, Switch7/3, Add3/2  "Signal 3"
  Mux/1 -> Scope/1
  Mux1/1 -> Scope/2
  Mux2/1 -> Scope/3
  Mux3/1 -> Scope/4
  Switch1/1 -> Add1/1, Mux1/1  "Bruit canal 1"
  Add4/1 -> Product/2
  Add/1 -> Switch4/1
  Constant4/1 -> Switch4/2
  Add5/1 -> Product1/1
  Constant5/1 -> Switch5/2
  Add1/1 -> Switch5/1
  Constant6/1 -> Switch6/2
  Add2/1 -> Switch6/1
  Constant7/1 -> Switch7/2
  Add3/1 -> Switch7/1
  Add7/1 -> Product3/1
  Product/1 -> Round/1
  Product1/1 -> Round1/1
  Constant12/1 -> Product/1
  Product2/1 -> Round2/1
  Add6/1 -> Product2/2
  Constant15/1 -> Product3/2
  Product3/1 -> Round3/1
  Constant8/1 -> Add4/1
  Switch4/1 -> Add4/2
  Constant9/1 -> Add5/1
  Constant13/1 -> Product1/2
  Switch5/1 -> Add5/2
  Constant14/1 -> Product2/1
  Constant10/1 -> Add6/1
  Switch6/1 -> Add6/2
  Constant11/1 -> Add7/1
  Switch7/1 -> Add7/2
  Round/1 -> Scope1/1, Signal Hydro Ref/1, Scope/5  "CAN Hydro Ref"
  Round1/1 -> Signal Hydro 1/1, Scope/6  "CAN Hydro 1"
  Round2/1 -> Signal Hydro 2/1, Scope/7  "CAN Hydro 2"
  Round3/1 -> Signal Hydro 3/1, Scope/8  "CAN Hydro 3"
  From Workspace/1 -> Product4/2  "Signal ref"
  Discrete Pulse Generator/1 -> Product4/1
  Discrete Pulse Generator1/1 -> Product5/1
  From Workspace1/1 -> Product5/2  "Signal 1"
  From Workspace2/1 -> Product6/2  "Signal 2"
  Discrete Pulse Generator2/1 -> Product6/1
  Discrete Pulse Generator3/1 -> Product7/1
  From Workspace3/1 -> Product7/2  "Signal 3"

== system Simulation_DOA_rearanged_2020a/Subsystem2 ==
  In1 : Inport
  Enable : EnablePort
  Array Plot : ArrayPlot
  Buffer1 : Buffer  N=FFT_LENGTH  OutputFrames=off
  wires:
  Buffer1/1 -> Array Plot/1
  In1/1 -> Buffer1/1

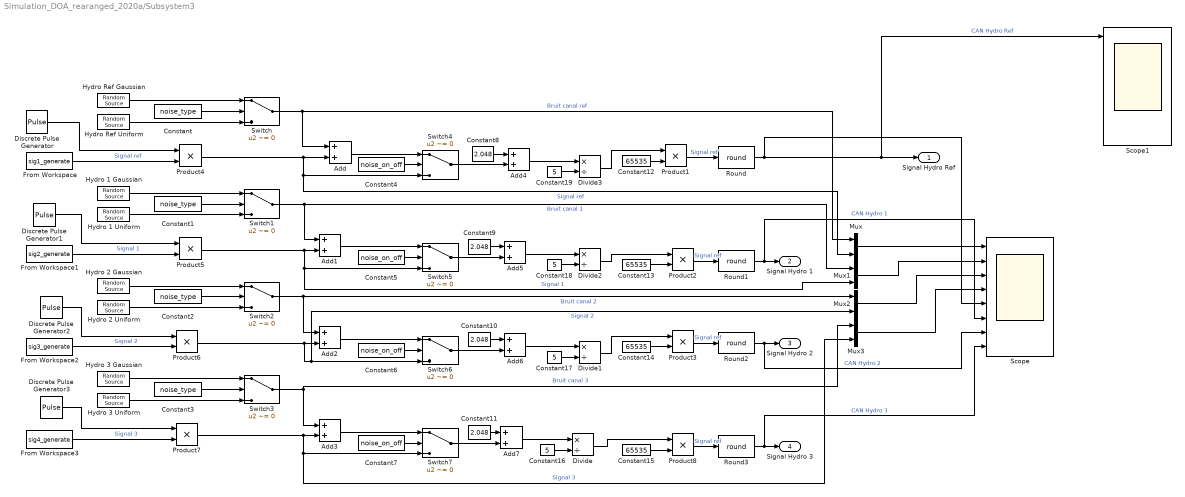
== system Simulation_DOA_rearanged_2020a/Subsystem3 ==
  Add{,1..7} (8 alike) : Sum
  Constant{,1..3} (4 alike) : Constant  Value=noise_type  VectorParams1D=off  SampleTime=-1
  Constant{8..11} (4 alike) : Constant  Value=2.048  VectorParams1D=off  SampleTime=-1
  Constant{12..15} (4 alike) : Constant  Value=65535  SampleTime=-1
  Constant{16..19} (4 alike) : Constant  Value=5  SampleTime=-1
  Constant{4..7} (4 alike) : Constant  Value=noise_on_off  VectorParams1D=off  SampleTime=-1
  Discrete Pulse Generator{,1..3} (4 alike) : DiscretePulseGenerator  Period=256  PulseWidth=128  SampleTime=1/Sampling_rate
  Divide{,1..3} (4 alike) : Product  Inputs=*/
  From Workspace : FromWorkspace  VariableName=sig1_generate  SampleTime=1/Sampling_rate
  From Workspace1 : FromWorkspace  VariableName=sig2_generate  SampleTime=1/Sampling_rate
  From Workspace2 : FromWorkspace  VariableName=sig3_generate  SampleTime=1/Sampling_rate
  From Workspace3 : FromWorkspace  VariableName=sig4_generate  SampleTime=1/Sampling_rate
  Hydro 1 Gaussian : dspsrcs4/Random Source  SrcType=Gaussian  NormMethod=Ziggurat  CltLength=12  MinVal=0  MaxVal=1  MeanVal=0  VarVal=variance  RepMode=Specify seed  rawSeed=randSeed2  IsInherit=off  SampMode=Discrete  SampTime=1/Sampling_rate  SampFrame=1  DataType=Double  OutComplex=Real  OutputFrames=off
  Hydro 1 Uniform : dspsrcs4/Random Source  SrcType=Uniform  NormMethod=Ziggurat  CltLength=12  MinVal=-0.9  MaxVal=0.9  MeanVal=0  VarVal=1  RepMode=Specify seed  rawSeed=4948745  IsInherit=off  SampMode=Discrete  SampTime=1/Sampling_rate  SampFrame=1  DataType=Double  OutComplex=Real  OutputFrames=off
  Hydro 2 Gaussian : dspsrcs4/Random Source  SrcType=Gaussian  NormMethod=Ziggurat  CltLength=12  MinVal=0  MaxVal=1  MeanVal=0  VarVal=variance  RepMode=Specify seed  rawSeed=randSeed3  IsInherit=off  SampMode=Discrete  SampTime=1/Sampling_rate  SampFrame=1  DataType=Double  OutComplex=Real  OutputFrames=off
  Hydro 2 Uniform : dspsrcs4/Random Source  SrcType=Uniform  NormMethod=Ziggurat  CltLength=12  MinVal=-0.9  MaxVal=0.9  MeanVal=0  VarVal=1  RepMode=Specify seed  rawSeed=2398385  IsInherit=off  SampMode=Discrete  SampTime=1/Sampling_rate  SampFrame=1  DataType=Double  OutComplex=Real  OutputFrames=off
  Hydro 3 Gaussian : dspsrcs4/Random Source  SrcType=Gaussian  NormMethod=Ziggurat  CltLength=12  MinVal=0  MaxVal=1  MeanVal=0  VarVal=variance  RepMode=Specify seed  rawSeed=randSeed4  IsInherit=off  SampMode=Discrete  SampTime=1/Sampling_rate  SampFrame=1  DataType=Double  OutComplex=Real  OutputFrames=off
  Hydro 3 Uniform : dspsrcs4/Random Source  SrcType=Uniform  NormMethod=Ziggurat  CltLength=12  MinVal=-0.9  MaxVal=0.9  MeanVal=0  VarVal=1  RepMode=Specify seed  rawSeed=9274563  IsInherit=off  SampMode=Discrete  SampTime=1/Sampling_rate  SampFrame=1  DataType=Double  OutComplex=Real  OutputFrames=off
  Hydro Ref Gaussian : dspsrcs4/Random Source  SrcType=Gaussian  NormMethod=Ziggurat  CltLength=12  MinVal=0  MaxVal=1  MeanVal=0  VarVal=variance  RepMode=Specify seed  rawSeed=randSeed1  IsInherit=off  SampMode=Discrete  SampTime=1/Sampling_rate  SampFrame=1  DataType=Double  OutComplex=Real  OutputFrames=off
  Hydro Ref Uniform : dspsrcs4/Random Source  SrcType=Uniform  NormMethod=Ziggurat  CltLength=12  MinVal=-0.9  MaxVal=0.9  MeanVal=0  VarVal=1  RepMode=Specify seed  rawSeed=3409859  IsInherit=off  SampMode=Discrete  SampTime=1/Sampling_rate  SampFrame=1  DataType=Double  OutComplex=Real  OutputFrames=off
  Mux{,1..3} (4 alike) : Mux  Inputs=2
  Product{1..8} (8 alike) : Product
  Round{,1..3} (4 alike) : Rounding  Operator=round
  Scope : Scope  NumInputPorts=8
  Scope1 : Scope  NumInputPorts=8
  Switch{,1..7} (8 alike) : Switch  Criteria=u2 ~= 0
  Signal Hydro Ref : Outport
  Signal Hydro 1 : Outport  Port=2
  Signal Hydro 2 : Outport  Port=3
  Signal Hydro 3 : Outport  Port=4
  wires:
  Hydro Ref Uniform/1 -> Switch/3
  Hydro Ref Gaussian/1 -> Switch/1
  Product4/1 -> Switch4/3, Mux/2, Add/2  "Signal ref"
  Switch/1 -> Add/1, Mux/1  "Bruit canal ref"
  Constant/1 -> Switch/2
  Hydro 1 Uniform/1 -> Switch1/3
  Hydro 1 Gaussian/1 -> Switch1/1
  Constant1/1 -> Switch1/2
  Product5/1 -> Switch5/3, Mux1/2, Add1/2  "Signal 1"
  Switch2/1 -> Add2/1, Mux2/1  "Bruit canal 2"
  Hydro 2 Uniform/1 -> Switch2/3
  Hydro 2 Gaussian/1 -> Switch2/1
  Constant2/1 -> Switch2/2
  Product6/1 -> Switch6/3, Mux2/2, Add2/2  "Signal 2"
  Switch3/1 -> Mux3/1, Add3/1  "Bruit canal 3"
  Hydro 3 Uniform/1 -> Switch3/3
  Hydro 3 Gaussian/1 -> Switch3/1
  Constant3/1 -> Switch3/2
  Product7/1 -> Mux3/2, Switch7/3, Add3/2  "Signal 3"
  Mux/1 -> Scope/1
  Mux1/1 -> Scope/2
  Mux2/1 -> Scope/3
  Mux3/1 -> Scope/4
  Switch1/1 -> Add1/1, Mux1/1  "Bruit canal 1"
  Add/1 -> Switch4/1
  Constant4/1 -> Switch4/2
  Constant5/1 -> Switch5/2
  Add1/1 -> Switch5/1
  Constant6/1 -> Switch6/2
  Add2/1 -> Switch6/1
  Constant7/1 -> Switch7/2
  Add3/1 -> Switch7/1
  Constant8/1 -> Add4/1
  Switch4/1 -> Add4/2
  Constant9/1 -> Add5/1
  Switch5/1 -> Add5/2
  Constant10/1 -> Add6/1
  Switch6/1 -> Add6/2
  Constant11/1 -> Add7/1
  Switch7/1 -> Add7/2
  Round/1 -> Scope1/1, Signal Hydro Ref/1, Scope/5  "CAN Hydro Ref"
  Round1/1 -> Signal Hydro 1/1, Scope/6  "CAN Hydro 1"
  Round2/1 -> Signal Hydro 2/1, Scope/7  "CAN Hydro 2"
  Round3/1 -> Signal Hydro 3/1, Scope/8  "CAN Hydro 3"
  From Workspace/1 -> Product4/2  "Signal ref"
  Discrete Pulse Generator/1 -> Product4/1
  Discrete Pulse Generator1/1 -> Product5/1
  From Workspace1/1 -> Product5/2  "Signal 1"
  From Workspace2/1 -> Product6/2  "Signal 2"
  Discrete Pulse Generator2/1 -> Product6/1
  Discrete Pulse Generator3/1 -> Product7/1
  From Workspace3/1 -> Product7/2  "Signal 3"
  Product1/1 -> Round/1  "Signal ref"
  Product3/1 -> Round2/1  "Signal ref"
  Product8/1 -> Round3/1  "Signal ref"
  Constant12/1 -> Product1/2
  Constant13/1 -> Product2/2
  Constant14/1 -> Product3/2
  Constant15/1 -> Product8/2
  Divide/1 -> Product8/1
  Constant16/1 -> Divide/2
  Add7/1 -> Divide/1
  Divide3/1 -> Product1/1
  Constant19/1 -> Divide3/2
  Add4/1 -> Divide3/1
  Constant18/1 -> Divide2/2
  Add5/1 -> Divide2/1
  Divide2/1 -> Product2/1
  Divide1/1 -> Product3/1
  Constant17/1 -> Divide1/2
  Add6/1 -> Divide1/1
  Product2/1 -> Round1/1  "Signal ref"

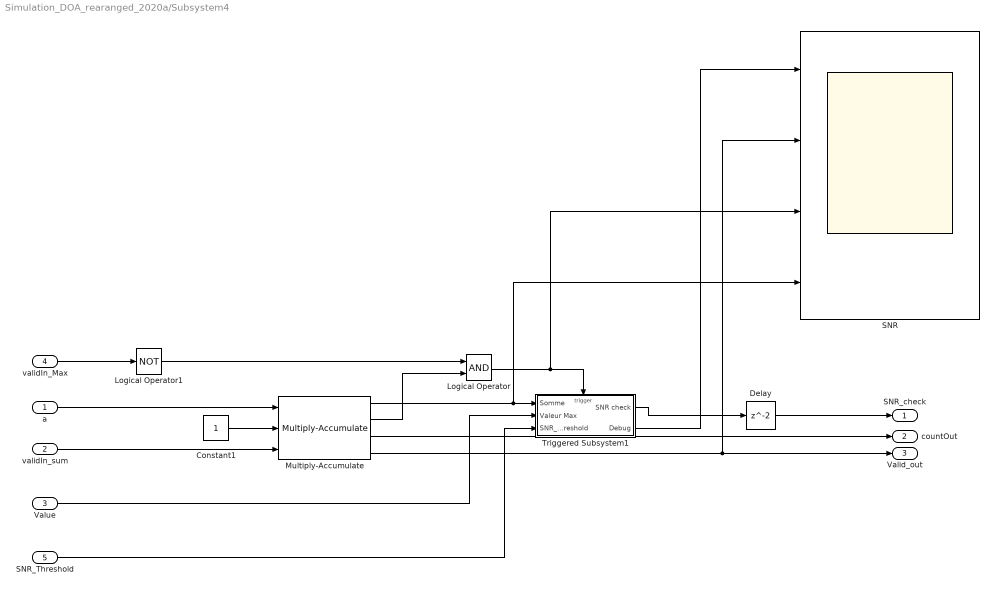
== system Simulation_DOA_rearanged_2020a/Subsystem4 ==
  a : Inport
  validIn_sum : Inport  Port=2
  " Value" : Inport  Port=3
  validIn_Max : Inport  Port=4
  SNR_Threshold : Inport  Port=5
  Constant1 : Constant  OutDataTypeStr=fixdt(1,27,8)  SampleTime=1/256000
  Delay : Delay
  Logical Operator : Logic  AllPortsSameDT=off  OutDataTypeStr=boolean
  Logical Operator1 : Logic  Operator=NOT  AllPortsSameDT=off  OutDataTypeStr=boolean
  Multiply-Accumulate : hdlsllib/HDL Operations/Multiply-Accumulate  opMode=Streaming - using Number of Samples  initValueSetting=Dialog  initValue=0  initValueSetting2=Dialog  initValue2=0  initValueSetting3=Dialog  initValue3=0  num_samples=256  RndMeth2=Floor  RndMeth3=Floor  datatype2=Inherit: Inherit via back propagation  datatype3=fixdt(1,27,8)  validOut=on  endInandOut=on  startOut=on  countOut=on  dim=-1  DoSatur=off  parallel=off
      settings: SourceProductBaseCode=SL
  SNR : Scope  NumInputPorts=4
  Triggered Subsystem1 : Subsystem  TreatAsAtomicUnit=on
  SNR_check : Outport
  countOut : Outport  Port=2
  Valid_out : Outport  Port=3
  wires:
  validIn_sum/1 -> Multiply-Accumulate/3
  Constant1/1 -> Multiply-Accumulate/2
  Multiply-Accumulate/1 -> SNR/4, Triggered Subsystem1/1(Somme)
  " Value"/1 -> Triggered Subsystem1/2(" Valeur Max")
  Triggered Subsystem1/1(SNR check) -> Delay/1
  Multiply-Accumulate/3 -> countOut/1
  validIn_Max/1 -> Logical Operator1/1
  Logical Operator1/1 -> Logical Operator/1
  Multiply-Accumulate/2 -> Logical Operator/2
  Multiply-Accumulate/4 -> SNR/2, Valid_out/1
  a/1 -> Multiply-Accumulate/1
  Logical Operator/1 -> SNR/3, Triggered Subsystem1/Trigger
  Delay/1 -> SNR_check/1
  Triggered Subsystem1/2(Debug) -> SNR/1
  SNR_Threshold/1 -> Triggered Subsystem1/3(SNR_Threshold)

== system Simulation_DOA_rearanged_2020a/Maximum Hydro 1/Subsystem ==
  Enable/Reset : Inport
  Add : Sum
  Data Type Conversion1 : DataTypeConversion  OutDataTypeStr=uint16  RndMeth=Nearest
  Delay : Delay  DelayLength=1  InitialCondition=0  UseCircularBuffer=on
  Product2 : Product
  Count : Outport  VectorParamsAs1DForOutWhenUnconnected=off
  wires:
  Enable/Reset/1 -> Add/1, Product2/1
  Add/1 -> Product2/2
  Delay/1 -> Count/1, Data Type Conversion1/1
  Product2/1 -> Delay/1
  Data Type Conversion1/1 -> Add/2

== system Simulation_DOA_rearanged_2020a/Maximum Hydro 2/Subsystem ==
  Enable/Reset : Inport
  Add : Sum
  Data Type Conversion1 : DataTypeConversion  OutDataTypeStr=uint16  RndMeth=Nearest
  Delay : Delay  DelayLength=1  InitialCondition=0  UseCircularBuffer=on
  Product2 : Product
  Count : Outport  VectorParamsAs1DForOutWhenUnconnected=off
  wires:
  Enable/Reset/1 -> Add/1, Product2/1
  Add/1 -> Product2/2
  Delay/1 -> Count/1, Data Type Conversion1/1
  Product2/1 -> Delay/1
  Data Type Conversion1/1 -> Add/2

== system Simulation_DOA_rearanged_2020a/Maximum Hydro 3/Subsystem ==
  Enable/Reset : Inport
  Add : Sum
  Data Type Conversion1 : DataTypeConversion  OutDataTypeStr=uint16  RndMeth=Nearest
  Delay : Delay  DelayLength=1  InitialCondition=0  UseCircularBuffer=on
  Product2 : Product
  Count : Outport  VectorParamsAs1DForOutWhenUnconnected=off
  wires:
  Enable/Reset/1 -> Add/1, Product2/1
  Add/1 -> Product2/2
  Delay/1 -> Count/1, Data Type Conversion1/1
  Product2/1 -> Delay/1
  Data Type Conversion1/1 -> Add/2

== system Simulation_DOA_rearanged_2020a/Maximum Hydro Ref/Subsystem ==
  Enable/Reset : Inport
  Add : Sum
  Data Type Conversion1 : DataTypeConversion  OutDataTypeStr=uint16  RndMeth=Nearest
  Delay : Delay  DelayLength=1  InitialCondition=0  UseCircularBuffer=on
  Product2 : Product
  Count : Outport  VectorParamsAs1DForOutWhenUnconnected=off
  wires:
  Enable/Reset/1 -> Add/1, Product2/1
  Add/1 -> Product2/2
  Delay/1 -> Count/1, Data Type Conversion1/1
  Product2/1 -> Delay/1
  Data Type Conversion1/1 -> Add/2

== system Simulation_DOA_rearanged_2020a/Maximum Hydro Ref/Subsystem1 ==
  Trigger : Inport
  Input : Inport  Port=2
  Sample and Hold : dspsigops/Sample and Hold  trig=Falling edge  initCond=0  latchinput=off
  " " : Outport
  wires:
  Input/1 -> Sample and Hold/1
  Trigger/1 -> Sample and Hold/Trigger
  Sample and Hold/1 -> " "/1

== system Simulation_DOA_rearanged_2020a/Maximum Hydro Ref/Subsystem2 ==
  Trigger : Inport
  Input : Inport  Port=2
  Sample and Hold : dspsigops/Sample and Hold  trig=Falling edge  initCond=0  latchinput=off
  " " : Outport
  wires:
  Input/1 -> Sample and Hold/1
  Trigger/1 -> Sample and Hold/Trigger
  Sample and Hold/1 -> " "/1

== system Simulation_DOA_rearanged_2020a/Maximum Hydro Ref/Subsystem3 ==
  Trigger : Inport
  Input : Inport  Port=2
  Sample and Hold : dspsigops/Sample and Hold  trig=Falling edge  initCond=0  latchinput=off
  " " : Outport
  wires:
  Input/1 -> Sample and Hold/1
  Trigger/1 -> Sample and Hold/Trigger
  Sample and Hold/1 -> " "/1

== system Simulation_DOA_rearanged_2020a/Maximum Hydro Ref/Subsystem4 ==
  Trigger : Inport
  Input : Inport  Port=2
  Sample and Hold : dspsigops/Sample and Hold  trig=Falling edge  initCond=0  latchinput=off
  " " : Outport
  wires:
  Input/1 -> Sample and Hold/1
  Trigger/1 -> Sample and Hold/Trigger
  Sample and Hold/1 -> " "/1

== system Simulation_DOA_rearanged_2020a/Maximum Hydro Ref/Subsystem5 ==
  Trigger : Inport
  Input : Inport  Port=2
  Sample and Hold : dspsigops/Sample and Hold  trig=Falling edge  initCond=0  latchinput=off
  " " : Outport
  wires:
  Input/1 -> Sample and Hold/1
  Trigger/1 -> Sample and Hold/Trigger
  Sample and Hold/1 -> " "/1

== system Simulation_DOA_rearanged_2020a/Maximum Hydro Ref/Subsystem6 ==
  Trigger : Inport
  Input : Inport  Port=2
  Sample and Hold : dspsigops/Sample and Hold  trig=Falling edge  initCond=0  latchinput=off
  " " : Outport
  wires:
  Input/1 -> Sample and Hold/1
  Trigger/1 -> Sample and Hold/Trigger
  Sample and Hold/1 -> " "/1
